simulink model "Project_2_Kinematic_Model"  (R2025a)
settings: Solver=VariableStepAuto  StartTime=0.0  StopTime=1000  RelTol=1e-3
undefined symbols (not defined in the file or in its folder): carData
settings Model: Creator=jr843  LastModifiedBy=jr843

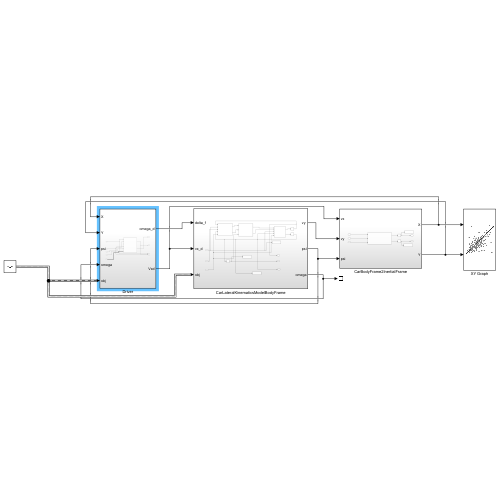
[thumbnail: Simulink's stored preview of the top-level diagram]
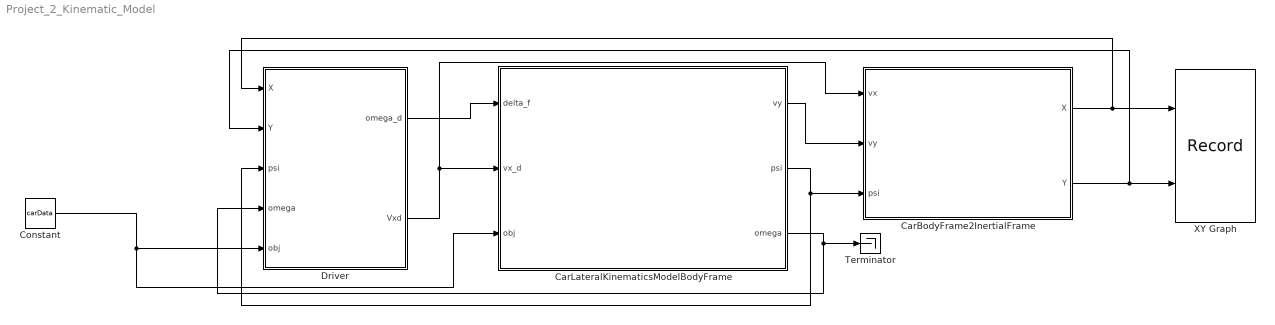
== system Project_2_Kinematic_Model ==
  CarBodyFrame2InertialFrame : Subsystem
  CarLateralKinematicsModelBodyFrame : Subsystem
  Constant : Constant  Value=carData  OutDataTypeStr=Bus: slBus1
  Driver : Subsystem
  Terminator : Terminator
  XY Graph : Record  NumPorts=2.0  FileSettingsInternal="{\"entries\":[{\"content\":{\"excelSettings\":{\"content\":{},\"type\":\"Streamout.ExcelSettings\"},\"parquetSettings\":{\"content\":{},\"type\":\"Streamout.ParquetSettings\"}},\"type\":\"Streamout.FileSettingStorage\",\"uuid\":\"\"}],\"packageUris\":[\"http:\\/\\/schema.mathworks.com\\/mf0\\/streamout_blocks\\/R2020a\"],\"version\":\"1.0\"}"  FrameSettings=[0, 0]  Layout=[1 1]  SignalsInternal="{\"entries\":[{\"content\":{\"signals\":[{\"content\":{\"blockPath\":[],\"dimensions\":[1],\"domain\":\"\",\"lineColor\":\"#a2142f\",\"plots\":[ 1 ],\"port\":1,\"sid\":[\"\"],\"signalID\":1,\"signalName\":\"CarBodyFrame2InertialFrame:1\"},\"type\":\"RecordBlkView.Signal\",\"uuid\":\"\"},{\"content\":{\"blockPath\":[],\"dimensions\":[1],\"domain\":\"\",\"lineColor\":\"#139fff\",\"plots\":[ 1 ],\"port\":2,\"sid\":[\"\"],\"signalID\":2,\"signalName\":\"CarBodyFrame2InertialFrame:2\"},\"type\":\"RecordBlkView.Signal\",\"uuid\":\"\"}]},\"type\":\"RecordBlkView.InputSignals\",\"uuid\":\"\"}],\"packageUris\":[\"http:\\/\\/schema.mathworks.com\\/mf0\\/streamout_blocks\\/R2020a\"],\"version\":\"1.0\"}"  VisualizationBindings="{\"xyplotplugin\":{\"info\":[{\"series\":[{\"bindingParametersList\":[{\"parameter\":\"X-Axis\",\"signalID\":1,\"signalName\":\"CarBodyFrame2InertialFrame:1\"},{\"parameter\":\"Y-Axis\",\"signalID\":2,\"signalName\":\"CarBodyFrame2InertialFrame:2\"}],\"seriesID\":0}],\"subplotID\":1}]}}"  CompatibilityTag=XY  st=-1
  wires:
  Driver/1(omega_d) -> CarLateralKinematicsModelBodyFrame/1(delta_f)
  CarLateralKinematicsModelBodyFrame/3(omega) -> Driver/4(omega), Terminator/1
  Driver/2(Vxd) -> CarBodyFrame2InertialFrame/1(vx), CarLateralKinematicsModelBodyFrame/2("vx_d ")
  CarBodyFrame2InertialFrame/1(X) -> Driver/1(X), XY Graph/1
  CarLateralKinematicsModelBodyFrame/2(psi) -> Driver/3(psi), CarBodyFrame2InertialFrame/3(psi)
  CarBodyFrame2InertialFrame/2(Y) -> Driver/2(Y), XY Graph/2
  CarLateralKinematicsModelBodyFrame/1("vy ") -> CarBodyFrame2InertialFrame/2(vy)
  Constant/1 -> CarLateralKinematicsModelBodyFrame/3(obj), Driver/5(obj)

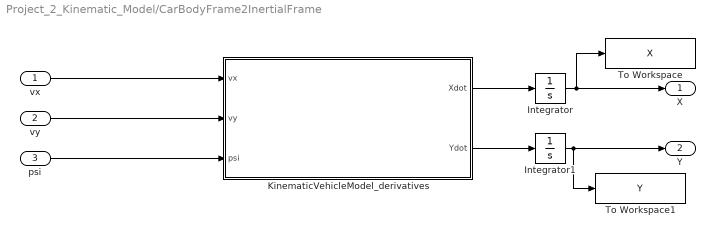
== system Project_2_Kinematic_Model/CarBodyFrame2InertialFrame ==
  vx : Inport
  vy : Inport  Port=2
  psi : Inport  Port=3
  Integrator : Integrator  InitialCondition=carData.init.X0
  Integrator1 : Integrator  InitialCondition=carData.init.Y0
  KinematicVehicleModel_derivatives : MATLAB Function  TreatAsAtomicUnit=on
  To Workspace : ToWorkspace  VariableName=X  SaveFormat=Timeseries  SampleTime=-1
  To Workspace1 : ToWorkspace  VariableName=Y  SaveFormat=Timeseries  SampleTime=-1
  X : Outport
  Y : Outport  Port=2
  wires:
  KinematicVehicleModel_derivatives/1(Xdot) -> Integrator/1
  KinematicVehicleModel_derivatives/2(Ydot) -> Integrator1/1
  Integrator/1 -> To Workspace/1, X/1
  Integrator1/1 -> To Workspace1/1, Y/1
  vx/1 -> KinematicVehicleModel_derivatives/1(vx)
  vy/1 -> KinematicVehicleModel_derivatives/2(vy)
  psi/1 -> KinematicVehicleModel_derivatives/3(psi)

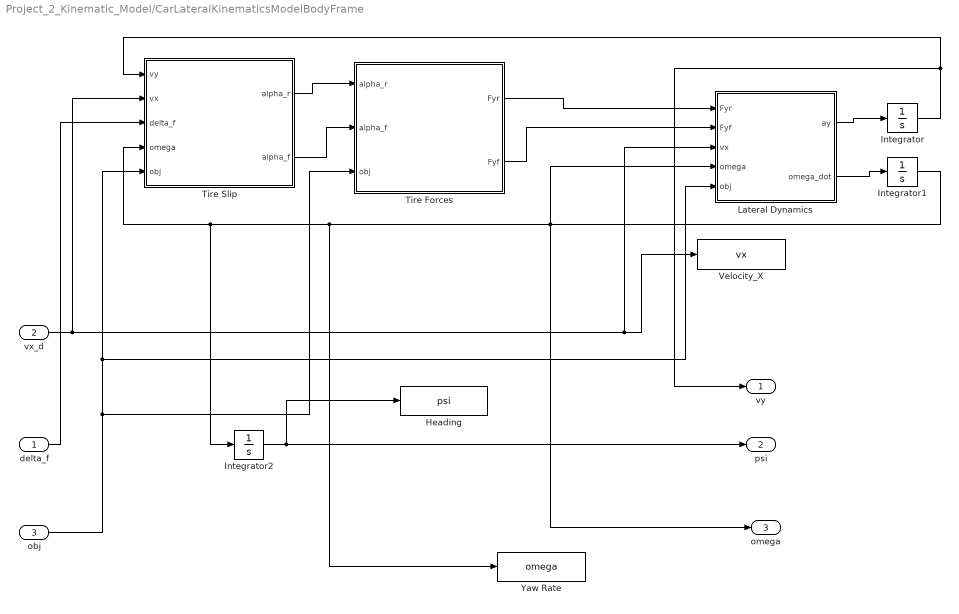
== system Project_2_Kinematic_Model/CarLateralKinematicsModelBodyFrame ==
  delta_f : Inport
  "vx_d " : Inport  Port=2
  obj : Inport  Port=3
  Heading : ToWorkspace  VariableName=psi  SaveFormat=Timeseries  SampleTime=-1
  Integrator : Integrator
  Integrator1 : Integrator
  Integrator2 : Integrator
  Lateral Dynamics : MATLAB Function  TreatAsAtomicUnit=on
  Tire Forces : MATLAB Function  TreatAsAtomicUnit=on
  Tire Slip : MATLAB Function  TreatAsAtomicUnit=on
  Velocity_X : ToWorkspace  VariableName=vx  SaveFormat=Timeseries  SampleTime=-1
  Yaw Rate : ToWorkspace  VariableName=omega  SaveFormat=Timeseries  SampleTime=-1
  "vy " : Outport
  psi : Outport  Port=2
  omega : Outport  Port=3
  wires:
  Integrator2/1 -> psi/1, Heading/1
  "vx_d "/1 -> Tire Slip/2(vx), Velocity_X/1, Lateral Dynamics/3(vx)
  delta_f/1 -> Tire Slip/3(delta_f)
  Integrator/1 -> "vy "/1, Tire Slip/1(vy)
  Tire Slip/1(alpha_r) -> Tire Forces/1(alpha_r)
  Tire Slip/2(alpha_f) -> Tire Forces/2(alpha_f)
  Lateral Dynamics/1(ay) -> Integrator/1
  Lateral Dynamics/2(omega_dot) -> Integrator1/1
  Integrator1/1 -> omega/1, Lateral Dynamics/4(omega), Yaw Rate/1, Integrator2/1, Tire Slip/4(omega)
  Tire Forces/1(Fyr) -> Lateral Dynamics/1(Fyr)
  Tire Forces/2(Fyf) -> Lateral Dynamics/2(Fyf)
  obj/1 -> Tire Forces/3(obj), Lateral Dynamics/5(obj), Tire Slip/5(obj)

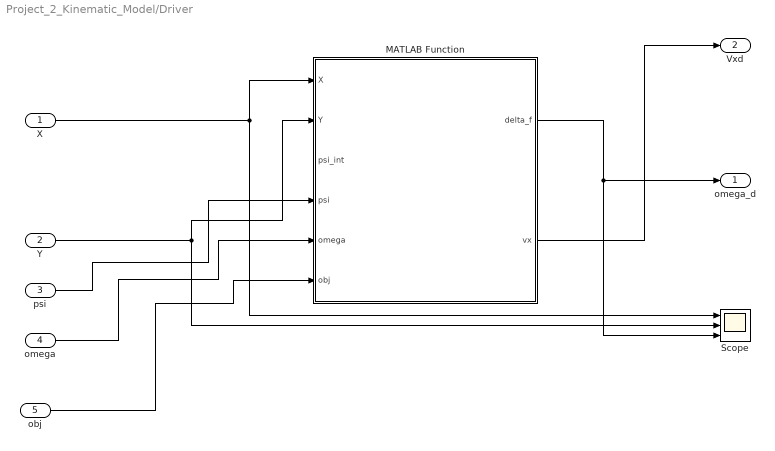
== system Project_2_Kinematic_Model/Driver ==
  X : Inport
  Y : Inport  Port=2
  psi : Inport  Port=3
  omega : Inport  Port=4
  obj : Inport  Port=5
  MATLAB Function : MATLAB Function  TreatAsAtomicUnit=on
  Scope : Scope  NumInputPorts=3
      settings: ActiveDisplayYMinimum=-351.50186  ActiveDisplayYMaximum=1255.09761
  omega_d : Outport
  Vxd : Outport  Port=2
  wires:
  MATLAB Function/1(delta_f) -> omega_d/1, Scope/3
  MATLAB Function/2(vx) -> Vxd/1
  X/1 -> Scope/1, MATLAB Function/1(X)
  Y/1 -> Scope/2, MATLAB Function/2(Y)
  psi/1 -> MATLAB Function/4(psi)
  omega/1 -> MATLAB Function/5(omega)
  obj/1 -> MATLAB Function/6(obj)

== matlab function Project_2_Kinematic_Model/CarLateralKinematicsModelBodyFrame/Tire Slip ==
  data: alpha_r output; vy input; alpha_f output; vx input; delta_f input; omega input; obj input
function [alpha_r, alpha_f]= fcn(vy, vx, delta_f, omega, obj)

if abs(vx) > obj.vx_threshold1
    alpha_f = delta_f - (vy + omega * obj.lf) / vx;
    alpha_r = - (vy - omega * obj.lr) / vx;

else
    alpha_f = 0;
    alpha_r = 0;

end

== matlab function Project_2_Kinematic_Model/CarLateralKinematicsModelBodyFrame/Tire Forces ==
  data: Fyr output; Fyf output; alpha_r input; alpha_f input; obj input
function [Fyr, Fyf] = fcn(alpha_r, alpha_f, obj)


Fyr = obj.Calpha_r * alpha_r;
Fyf = obj.Calpha_f * alpha_f;

if abs(Fyr) > obj.Fyrmax
    Fyr = obj.Fyrmax*sign(Fyr);

end

if abs(Fyf) > obj.Fyfmax
    Fyf = obj.Fyfmax*sign(Fyf);

end

== matlab function Project_2_Kinematic_Model/CarBodyFrame2InertialFrame/KinematicVehicleModel_derivatives ==
  data: vx input; vy input; psi input size=1; Xdot output; Ydot output
function [Xdot, Ydot] = fcn(vx, vy, psi)
    temp = TF(psi) * [vx;vy]; 
    Xdot = temp(1);
    Ydot = temp(2);
  
end

function y = TF(psi)
    y = [cos(psi), -sin(psi); sin(psi), cos(psi)];
end

== matlab function Project_2_Kinematic_Model/CarLateralKinematicsModelBodyFrame/Lateral Dynamics ==
  data: Fyr input; ay output; Fyf input; vx input; omega input; omega_dot output; obj input
function [ay, omega_dot]= fcn(Fyr, Fyf, vx, omega, obj)

ay = -vx * omega + (Fyf + Fyr)/obj.Mass;

omega_dot = (Fyf*obj.lf - Fyr*obj.lr)/obj.Inertia;

end

== matlab function Project_2_Kinematic_Model/Driver/MATLAB Function ==
  data: X input; Y input; psi_int input; psi input; omega input; delta_f output; vx output; obj input
function [delta_f, vx] = SimplestDriver(X, Y, psi_int, psi, omega, obj)
% PID steering using psi_int (integral of heading error) and omega (yaw rate)

% --- track geometry ---
R   = 200;      % radius (m)
Lst = 900;      % straight length (m)
y0  = 0;        % bottom straight
y1  = 400;      % top straight
cy  = 200;      % arc centers' y
cxL = 0;        % left arc center x
cxR = Lst;      % right arc center x

% --- controller parameters ---
% PID on heading: delta = delta_ff + Kp*e_psi + Ki*psi_int - Kd*(omega - omega_ref)
Kp = 1.2;        % proportional on heading error
Ki = 0.5;        % integral gain (psi_int already integrates e_psi)
Kd = 0.25;       % derivative gain (on yaw-rate error)
Kv = 20;

maxSteer = 0.5;  % [rad] steering saturation
vx = obj.vxd;    % vehicle longitudinal speed

% Defaults
psi_ref = 0;
kappa_ref = 0;   % desired curvature (+ left, - right)
delta_ff = 0;    % feed-forward steering

if X > Lst
    % -------- Right semicircle (center at cxR,cy), CCW from bottom to top --------
    % Tangent heading is phi + pi/2
    phi = atan2(Y - cy, X - cxR);
    psi_ref = phi + pi/2;
    kappa_ref = 1/R;           % CCW positive
    % Geometric + understeer feed-forward (kept from your original style)
    delta_ff = (obj.lf + obj.lr)*kappa_ref + obj.understeerCoeff * vx^2;

elseif X < 0
    % -------- Left semicircle (center at cxL,cy), CCW from top to bottom --------
    phi = atan2(Y - cy, X - cxL);
    psi_ref = phi + pi/2;
    kappa_ref = 1/R;           % CCW positive
    delta_ff = (obj.lf + obj.lr)*kappa_ref + obj.understeerCoeff * vx^2;

else
    % -------- Inside rectangle (straights) --------
    if abs(Y) <= (y1-y0)/2
        % Bottom straight: motion +x => heading 0
        psi_ref = 0;
        kappa_ref = 0;
        delta_ff = 0;e_psi = wrapToPi(psi_ref - psi);
        delta = delta_ff + Kp*e_psi + Ki*psi_int;
      
    else
        % Top straight: motion -x => heading pi (or -pi)
        psi_ref = pi;
        kappa_ref = 0;
        delta_ff = 0;e_psi = wrapToPi(psi_ref - psi);
        delta = delta_ff + Kp*e_psi + Ki*psi_int;
    end
end



% --- heading error (wrapped to [-pi, pi]) ---
e_psi = wrapToPi(psi_ref - psi)

% --- yaw-rate reference from curvature ---
omega_ref = kappa_ref * vx;

% --- PID law using your integral and derivative signals ---
% integral term: psi_int is assumed to be \int e_psi dt (maintained in Simulink)
% derivative term: use yaw-rate error (omega - omega_ref), subtract to damp
delta = delta_ff + Kp*e_psi + Ki*psi_int - Kd*(omega - omega_ref);

% --- speed control ---
vx = obj.vxd - Kv*(Kp*e_psi + Ki*psi_int - Kd*(omega - omega_ref))

% --- saturation ---
delta_f = min(max(delta, -maxSteer), maxSteer);

end

% ---------- helpers ----------
function ang = wrapToPi(ang)
% Wrap any angle to [-pi, pi]
ang = mod(ang + pi, 2*pi) - pi;
end
